simulink model "lab_1"  (R2020a)
settings: Solver=VariableStepAuto  StartTime=0.0  StopTime=10.0  RelTol=1e-3
settings Model: Creator=Administrator  LastModifiedBy=Administrator

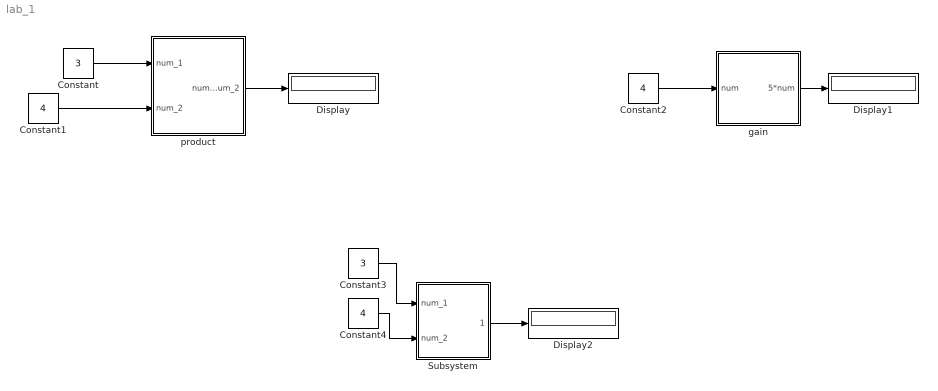
== system lab_1 ==
  Constant : Constant  Value=3
  Constant1 : Constant  Value=4
  Constant2 : Constant  Value=4
  Constant3 : Constant  Value=3
  Constant4 : Constant  Value=4
  Display : Display
  Display1 : Display
  Display2 : Display
  Subsystem : Subsystem
  gain : Subsystem
  product : Subsystem
  wires:
  Constant/1 -> product/1(num_1)
  Constant1/1 -> product/2(num_2)
  product/1(num_1*num_2) -> Display/1
  Constant2/1 -> gain/1(num)
  gain/1(5*num) -> Display1/1
  Subsystem/1(num_1+num_2) -> Display2/1
  Constant4/1 -> Subsystem/2(num_2)
  Constant3/1 -> Subsystem/1(num_1)

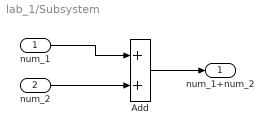
== system lab_1/Subsystem ==
  num_1 : Inport
  num_2 : Inport  Port=2
  Add : Sum
  num_1+num_2 : Outport
  wires:
  Add/1 -> num_1+num_2/1
  num_2/1 -> Add/2
  num_1/1 -> Add/1

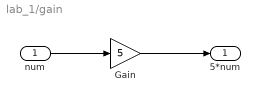
== system lab_1/gain ==
  num : Inport
  Gain : Gain  Gain=5
  5*num : Outport
  wires:
  Gain/1 -> 5*num/1
  num/1 -> Gain/1

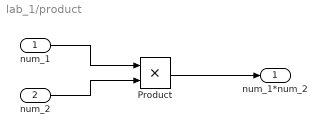
== system lab_1/product ==
  num_1 : Inport
  num_2 : Inport  Port=2
  Product : Product
  num_1*num_2 : Outport
  wires:
  num_2/1 -> Product/2
  num_1/1 -> Product/1
  Product/1 -> num_1*num_2/1
